simulink model "MotorDC"  (R2021a)
settings: Solver=ode4  StartTime=0.0  StopTime=0.4  FixedStep=0.001  RelTol=1e-3
values from neighbouring files (symbols this model uses):
  B = 0    [P1_script.m]    (also in simulacao1.m)
  J = 0.001    [P1_script.m]    (also in simulacao1.m = 0.00252)
  Kt = Te_rated/Ia_rated    (= 0.424752712124)    [P1_script.m]    (also in simulacao1.m)
  La = 1.7e-3    (= 0.0017)    [P1_script.m]    (also in simulacao1.m)
  Ra = 0.26    [P1_script.m]    (also in simulacao1.m)
settings Model: Creator=taylo  LastModifiedBy=taylo

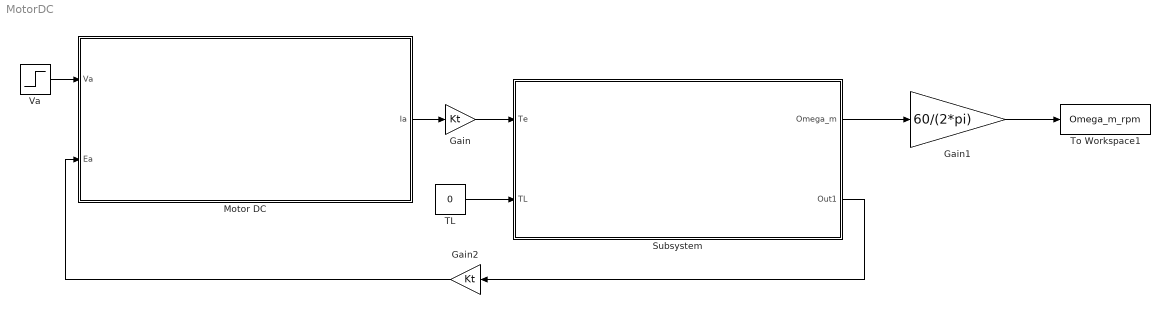
== system MotorDC ==
  Gain : Gain  Gain=Kt
  Gain1 : Gain  Gain=60/(2*pi)
  Gain2 : Gain  Gain=Kt
  Motor DC : Subsystem
  Subsystem : Subsystem
  TL : Constant  Value=0
  To Workspace1 : ToWorkspace  VariableName=Omega_m_rpm  SaveFormat=Timeseries  SampleTime=-1
  Va : Step  Time=0.05  After=70  SampleTime=0
  wires:
  Motor DC/1(Ia) -> Gain/1
  Gain/1 -> Subsystem/1(Te)
  TL/1 -> Subsystem/2(TL)
  Va/1 -> Motor DC/1(Va)
  Subsystem/1(Omega_m) -> Gain1/1
  Subsystem/2(Out1) -> Gain2/1
  Gain2/1 -> Motor DC/2(Ea)
  Gain1/1 -> To Workspace1/1

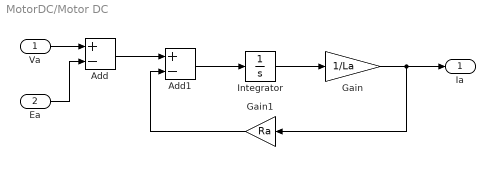
== system MotorDC/Motor DC ==
  Va : Inport
  Ea : Inport  Port=2
  Add : Sum  Inputs=+-
  Add1 : Sum  Inputs=+-
  Gain : Gain  Gain=1/La
  Gain1 : Gain  Gain=Ra
  Integrator : Integrator
  Ia : Outport
  wires:
  Add1/1 -> Integrator/1
  Gain1/1 -> Add1/2
  Add/1 -> Add1/1
  Va/1 -> Add/1
  Integrator/1 -> Gain/1
  Ea/1 -> Add/2
  Gain/1 -> Gain1/1, Ia/1

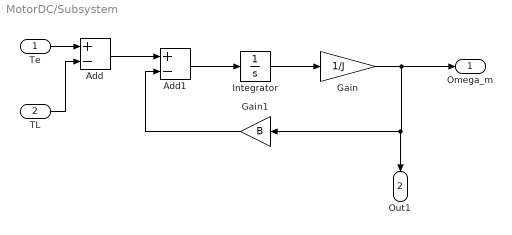
== system MotorDC/Subsystem ==
  Te : Inport
  TL : Inport  Port=2
  Add : Sum  Inputs=+-
  Add1 : Sum  Inputs=+-
  Gain : Gain  Gain=1/J
  Gain1 : Gain  Gain=B
  Integrator : Integrator
  Omega_m : Outport
  Out1 : Outport  Port=2
  wires:
  Te/1 -> Add/1
  Gain/1 -> Omega_m/1, Out1/1, Gain1/1
  Add/1 -> Add1/1
  TL/1 -> Add/2
  Add1/1 -> Integrator/1
  Gain1/1 -> Add1/2
  Integrator/1 -> Gain/1
